simulink model "PositionControl"  (R2019a)
settings: Solver=ode3  StartTime=0.0  StopTime=100.0  FixedStep=Ts  RelTol=1e-3
undefined symbols (not defined in the file): DiscIntNeverNeededParam, error_margin, Ts, w0, x0, y0
settings Model: Creator=mrblissfulgrin  LastModifiedBy=mrblissfulgrin
settings DataIOCC: ReturnWorkspaceOutputs=off

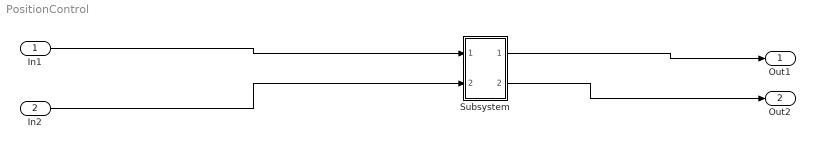
== system PositionControl ==
  In1 : Inport
  In2 : Inport  Port=2
  Subsystem : Subsystem
  Out1 : Outport
  Out2 : Outport  Port=2
  wires:
  In1/1 -> Subsystem/1(In1)
  In2/1 -> Subsystem/2(In2)
  Subsystem/1(Out1) -> Out1/1
  Subsystem/2(Out2) -> Out2/1

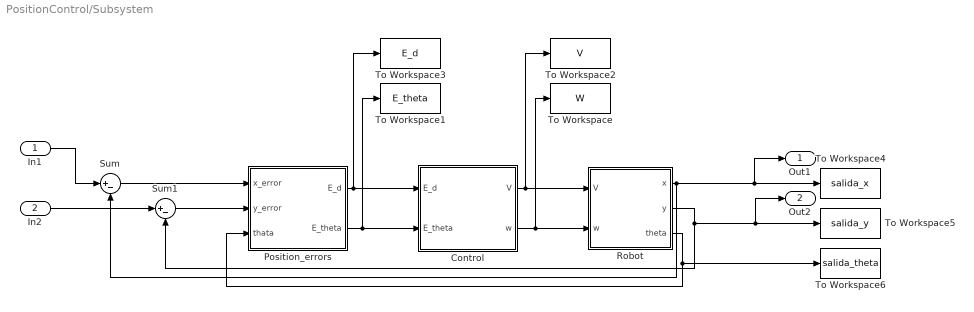
== system PositionControl/Subsystem ==
  In1 : Inport
  In2 : Inport  Port=2
  Control : Subsystem
  Position_errors : Subsystem
  Robot : Subsystem
  Sum : Sum  Inputs=|+-
  Sum1 : Sum  Inputs=|+-
  To Workspace : ToWorkspace  VariableName=W  SaveFormat=Structure With Time  SampleTime=Ts
  To Workspace1 : ToWorkspace  VariableName=E_theta  SaveFormat=Structure With Time  SampleTime=Ts
  To Workspace2 : ToWorkspace  VariableName=V  SaveFormat=Structure With Time  SampleTime=Ts
  To Workspace3 : ToWorkspace  VariableName=E_d  SaveFormat=Structure With Time  SampleTime=Ts
  To Workspace4 : ToWorkspace  VariableName=salida_x  SaveFormat=Structure With Time  SampleTime=Ts
  To Workspace5 : ToWorkspace  VariableName=salida_y  SaveFormat=Structure With Time  SampleTime=Ts
  To Workspace6 : ToWorkspace  VariableName=salida_theta  SaveFormat=Structure With Time  SampleTime=Ts
  Out1 : Outport
  Out2 : Outport  Port=2
  wires:
  In2/1 -> Sum1/1
  In1/1 -> Sum/1
  Robot/1(x) -> Out1/1, To Workspace4/1, Sum/2
  Robot/2(y) -> Out2/1, To Workspace5/1, Sum1/2
  Sum1/1 -> Position_errors/2(y_error)
  Position_errors/2(E_theta) -> To Workspace1/1, Control/2(E_theta)
  Position_errors/1(E_d) -> To Workspace3/1, Control/1(E_d)
  Control/1(V) -> To Workspace2/1, Robot/1(V)
  Sum/1 -> Position_errors/1(x_error)
  Robot/3(theta) -> To Workspace6/1, Position_errors/3(thata)
  Control/2(w) -> To Workspace/1, Robot/2(w)

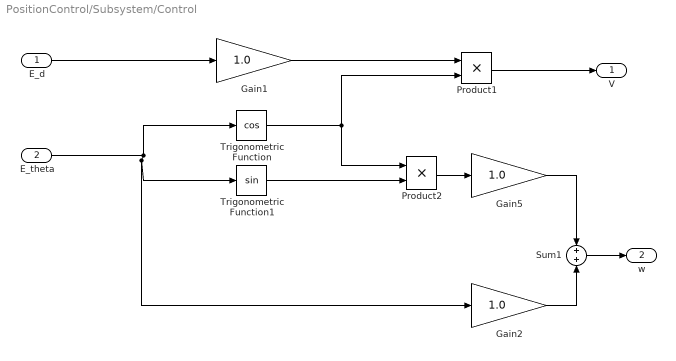
== system PositionControl/Subsystem/Control ==
  E_d : Inport
  E_theta : Inport  Port=2
  Gain1 : Gain  Gain=1.0
  Gain2 : Gain  Gain=1.0
  Gain5 : Gain  Gain=1.0
  Product1 : Product
  Product2 : Product
  Sum1 : Sum
  Trigonometric Function : Trigonometry  Operator=cos
  Trigonometric Function1 : Trigonometry
  V : Outport
  w : Outport  Port=2
  wires:
  E_theta/1 -> Trigonometric Function/1, Trigonometric Function1/1, Gain2/1
  E_d/1 -> Gain1/1
  Trigonometric Function/1 -> Product1/2, Product2/1
  Product1/1 -> V/1
  Trigonometric Function1/1 -> Product2/2
  Product2/1 -> Gain5/1
  Gain1/1 -> Product1/1
  Gain5/1 -> Sum1/1
  Gain2/1 -> Sum1/2
  Sum1/1 -> w/1

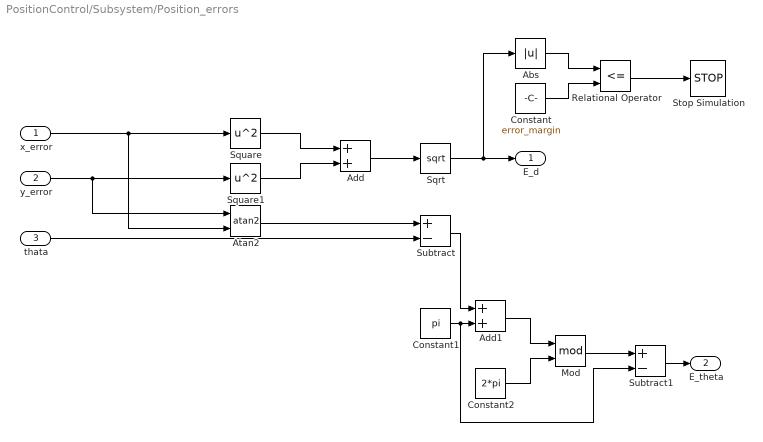
== system PositionControl/Subsystem/Position_errors ==
  x_error : Inport  SampleTime=Ts
  y_error : Inport  Port=2  SampleTime=Ts
  thata : Inport  Port=3  SampleTime=Ts
  Abs : Abs
  Add : Sum
  Add1 : Sum
  Atan2 : Trigonometry  Operator=atan2
  Constant : Constant  Value=error_margin  SampleTime=Ts
  Constant1 : Constant  Value=pi  SampleTime=Ts
  Constant2 : Constant  Value=2*pi
  Mod : Math  Operator=mod  SaturateOnIntegerOverflow=on
  Relational Operator : RelationalOperator  Operator=<=  OutDataTypeStr=boolean  RndMeth=Simplest
  Sqrt : Sqrt  SaturateOnIntegerOverflow=on
  Square : Math  Operator=square  SaturateOnIntegerOverflow=on
  Square1 : Math  Operator=square  SaturateOnIntegerOverflow=on
  Stop Simulation : Stop
  Subtract : Sum  Inputs=+-
  Subtract1 : Sum  Inputs=+-
  E_d : Outport  SampleTime=Ts
  E_theta : Outport  Port=2  SampleTime=Ts
  wires:
  Square/1 -> Add/1
  Sqrt/1 -> E_d/1, Abs/1
  y_error/1 -> Square1/1, Atan2/1
  Add/1 -> Sqrt/1
  Square1/1 -> Add/2
  thata/1 -> Subtract/2
  x_error/1 -> Square/1, Atan2/2
  Subtract/1 -> Add1/1
  Abs/1 -> Relational Operator/1
  Constant/1 -> Relational Operator/2
  Relational Operator/1 -> Stop Simulation/1
  Atan2/1 -> Subtract/1
  Constant1/1 -> Subtract1/2, Add1/2
  Add1/1 -> Mod/1
  Constant2/1 -> Mod/2
  Mod/1 -> Subtract1/1
  Subtract1/1 -> E_theta/1

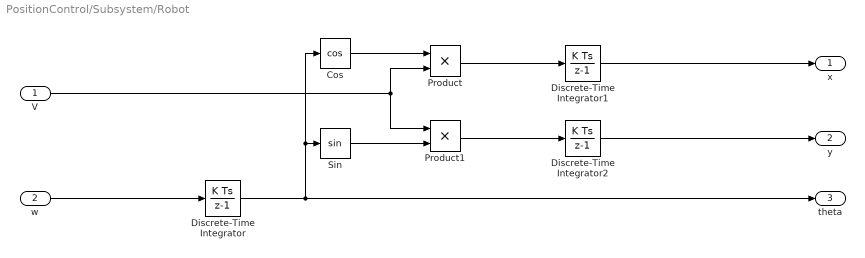
== system PositionControl/Subsystem/Robot ==
  V : Inport  SampleTime=Ts
  w : Inport  Port=2  SampleTime=Ts
  Cos : Trigonometry  Operator=cos
  Discrete-Time Integrator : DiscreteIntegrator  InitialCondition=w0  SampleTime=Ts  ICPrevOutput=DiscIntNeverNeededParam  ICPrevScaledInput=DiscIntNeverNeededParam
  Discrete-Time Integrator1 : DiscreteIntegrator  InitialCondition=x0  SampleTime=Ts  ICPrevOutput=DiscIntNeverNeededParam  ICPrevScaledInput=DiscIntNeverNeededParam
  Discrete-Time Integrator2 : DiscreteIntegrator  InitialCondition=y0  SampleTime=Ts  ICPrevOutput=DiscIntNeverNeededParam  ICPrevScaledInput=DiscIntNeverNeededParam
  Product : Product
  Product1 : Product
  Sin : Trigonometry
  x : Outport  SampleTime=Ts
  y : Outport  Port=2  SampleTime=Ts
  theta : Outport  Port=3  SampleTime=Ts
  wires:
  Discrete-Time Integrator2/1 -> y/1
  Product1/1 -> Discrete-Time Integrator2/1
  Cos/1 -> Product/1
  Sin/1 -> Product1/2
  w/1 -> Discrete-Time Integrator/1
  Discrete-Time Integrator1/1 -> x/1
  Product/1 -> Discrete-Time Integrator1/1
  V/1 -> Product/2, Product1/1
  Discrete-Time Integrator/1 -> theta/1, Sin/1, Cos/1
